simulink library "maddogLibrary"  (R2012b)
settings: Solver=ode45  StartTime=0.0  StopTime=10.0  RelTol=1e-3
libraries: xbsIndex_r4 x208, maddogLibrary x2
settings Model: Creator=tmadden  LastModifiedBy=tmadden

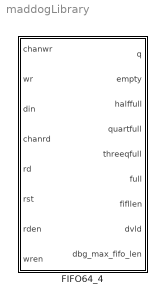
== system maddogLibrary ==
  FIFO64_4 : Subsystem  mask{fifo_len_p2=9}
      mask prompts: fifo_len_p2 "Fifo Len, (enter 8 for 256)"

== system maddogLibrary/FIFO64_4 ==
  chanwr : Inport
  wr : Inport  Port=2
  din : Inport  Port=3
  chanrd : Inport  Port=4
  rd : Inport  Port=5
  rst : Inport  Port=6
  rden : Inport  Port=7
  wren : Inport  Port=8
  FIFO32_1 : maddogLibrary/FIFO64_4/FIFO32_2
  FIFO32_2 : Subsystem
  Subsystem1 : Subsystem
  Subsystem2 : Subsystem
  q : Outport
  empty : Outport  Port=2
  halffull : Outport  Port=3
  quartfull : Outport  Port=4
  threeqfull : Outport  Port=5
  full : Outport  Port=6
  fifllen : Outport  Port=7
  dvld : Outport  Port=8
  dbg_max_fifo_len : Outport  Port=9
  wires:
  wr/1 -> FIFO32_1/2, FIFO32_2/2(wr)
  rst/1 -> FIFO32_1/6, FIFO32_2/6(rst)
  chanrd/1 -> Subsystem2/2(chanrd), Subsystem1/4(In4), FIFO32_1/4, FIFO32_2/4(chanrd)
  din/1 -> FIFO32_1/3, FIFO32_2/3(din)
  chanwr/1 -> Subsystem2/1(chanwr), FIFO32_1/1, FIFO32_2/1(chanwr)
  rd/1 -> FIFO32_1/5, FIFO32_2/5(rd)
  FIFO32_2/1(q) -> Subsystem1/1(In1)
  FIFO32_2/2(empty) -> Subsystem1/2(In2)
  FIFO32_2/3(halffull) -> Subsystem1/3(In3)
  FIFO32_2/4(quartfull) -> Subsystem1/5(In5)
  FIFO32_2/5(threeqfull) -> Subsystem1/6(In6)
  FIFO32_2/6(full) -> Subsystem1/7(In7)
  FIFO32_2/7(fifllen) -> Subsystem1/8(In8)
  FIFO32_2/8(dvld) -> Subsystem1/9(In9)
  FIFO32_1/1 -> Subsystem1/10(In10)
  FIFO32_1/2 -> Subsystem1/11(In11)
  FIFO32_1/3 -> Subsystem1/12(In12)
  FIFO32_1/4 -> Subsystem1/13(In13)
  FIFO32_1/5 -> Subsystem1/14(In14)
  FIFO32_1/6 -> Subsystem1/15(In15)
  FIFO32_1/8 -> Subsystem1/17(In17)
  Subsystem1/1(Out1) -> q/1
  Subsystem1/2(Out2) -> empty/1
  Subsystem1/3(Out3) -> halffull/1
  Subsystem1/4(Out4) -> quartfull/1
  Subsystem1/5(Out5) -> threeqfull/1
  Subsystem1/6(Out6) -> full/1
  Subsystem1/7(Out7) -> fifllen/1
  Subsystem1/8(Out8) -> dvld/1
  rden/1 -> Subsystem2/3(rden)
  wren/1 -> Subsystem2/4(wren)
  Subsystem2/2(rdl) -> FIFO32_2/7(rden)
  Subsystem2/3(wrh) -> FIFO32_1/8
  Subsystem2/1(wrl) -> FIFO32_2/8(wren)
  Subsystem2/4(rdh) -> FIFO32_1/7
  FIFO32_1/7 -> Subsystem1/16(In16)
  FIFO32_1/9 -> dbg_max_fifo_len/1

== system maddogLibrary/FIFO64_4/FIFO32_2 ==
  chanwr : Inport
  wr : Inport  Port=2
  din : Inport  Port=3
  chanrd : Inport  Port=4
  rd : Inport  Port=5
  rst : Inport  Port=6
  rden : Inport  Port=7
  wren : Inport  Port=8
  FIFO16Cir_1 : Subsystem
  FIFO16Cir_2 : maddogLibrary/FIFO64_4/FIFO32_2/FIFO16Cir_1
  Subsystem : Subsystem
  Subsystem1 : Subsystem
  q : Outport
  empty : Outport  Port=2
  halffull : Outport  Port=3
  quartfull : Outport  Port=4
  threeqfull : Outport  Port=5
  full : Outport  Port=6
  fifllen : Outport  Port=7
  dvld : Outport  Port=8
  dbg_max_fifo_len : Outport  Port=9
  wires:
  wr/1 -> FIFO16Cir_2/2, FIFO16Cir_1/2(wr)
  rst/1 -> FIFO16Cir_2/6, FIFO16Cir_1/6(rst)
  chanrd/1 -> Subsystem/2(chanrd), Subsystem1/4(In4), FIFO16Cir_2/4, FIFO16Cir_1/4(chanrd)
  din/1 -> FIFO16Cir_2/3, FIFO16Cir_1/3(din)
  chanwr/1 -> Subsystem/1(chanwr), FIFO16Cir_2/1, FIFO16Cir_1/1(chanwr)
  rd/1 -> FIFO16Cir_2/5, FIFO16Cir_1/5(rd)
  Subsystem/2(rdl) -> FIFO16Cir_1/7(rden)
  Subsystem/1(wrl) -> FIFO16Cir_1/8(wren)
  Subsystem/4(rdh) -> FIFO16Cir_2/7
  Subsystem/3(wrh) -> FIFO16Cir_2/8
  FIFO16Cir_1/1(q) -> Subsystem1/1(In1)
  FIFO16Cir_1/2(empty) -> Subsystem1/2(In2)
  FIFO16Cir_1/3(halffull) -> Subsystem1/3(In3)
  FIFO16Cir_1/4(quartfill) -> Subsystem1/5(In5)
  FIFO16Cir_1/5(threequartfull) -> Subsystem1/6(In6)
  FIFO16Cir_1/6(full) -> Subsystem1/7(In7)
  FIFO16Cir_1/7(fifolen) -> Subsystem1/8(In8)
  FIFO16Cir_1/8(dvld_out) -> Subsystem1/9(In9)
  FIFO16Cir_2/1 -> Subsystem1/10(In10)
  FIFO16Cir_2/2 -> Subsystem1/11(In11)
  FIFO16Cir_2/3 -> Subsystem1/12(In12)
  FIFO16Cir_2/4 -> Subsystem1/13(In13)
  FIFO16Cir_2/5 -> Subsystem1/14(In14)
  FIFO16Cir_2/6 -> Subsystem1/15(In15)
  FIFO16Cir_2/7 -> Subsystem1/16(In16)
  FIFO16Cir_2/8 -> Subsystem1/17(In17)
  Subsystem1/1(Out1) -> q/1
  Subsystem1/2(Out2) -> empty/1
  Subsystem1/3(Out3) -> halffull/1
  Subsystem1/4(Out4) -> quartfull/1
  Subsystem1/5(Out5) -> threeqfull/1
  Subsystem1/6(Out6) -> full/1
  Subsystem1/7(Out7) -> fifllen/1
  Subsystem1/8(Out8) -> dvld/1
  rden/1 -> Subsystem/3(rden)
  wren/1 -> Subsystem/4(wren)
  FIFO16Cir_2/9 -> dbg_max_fifo_len/1

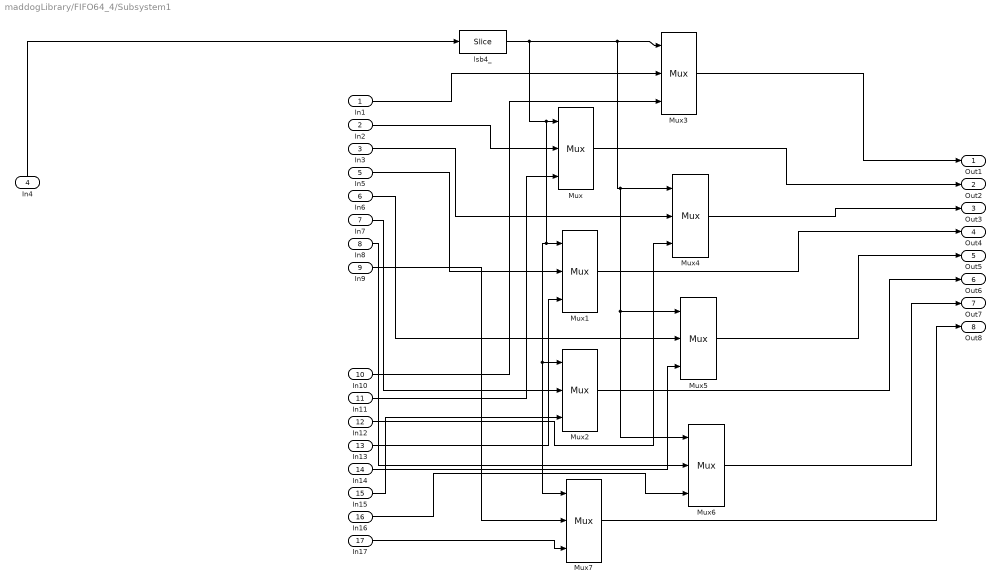
== system maddogLibrary/FIFO64_4/Subsystem1 ==
  In1 : Inport
  In2 : Inport  Port=2
  In3 : Inport  Port=3
  In4 : Inport  Port=4
  In5 : Inport  Port=5
  In6 : Inport  Port=6
  In7 : Inport  Port=7
  In8 : Inport  Port=8
  In9 : Inport  Port=9
  In10 : Inport  Port=10
  In11 : Inport  Port=11
  In12 : Inport  Port=12
  In13 : Inport  Port=13
  In14 : Inport  Port=14
  In15 : Inport  Port=15
  In16 : Inport  Port=16
  In17 : Inport  Port=17
  Mux{,1..7} (8 alike) : xbsIndex_r4/Mux  inputs=2  en=off  latency=0  precision=Full  arith_type=Unsigned  n_bits=16  bin_pt=14  quantization=Truncate  overflow=Wrap  dbl_ovrd=off  block_type=mux
  lsb4_ : xbsIndex_r4/Slice  nbits=1  boolean_output=on  mode=Lower Bit Location + Width  bit1=0  base1=MSB of Input  bit0=5  base0=LSB of Input  dbl_ovrd=off  block_type=slice
  Out1 : Outport
  Out2 : Outport  Port=2
  Out3 : Outport  Port=3
  Out4 : Outport  Port=4
  Out5 : Outport  Port=5
  Out6 : Outport  Port=6
  Out7 : Outport  Port=7
  Out8 : Outport  Port=8
  wires:
  In9/1 -> Mux7/2
  Mux3/1 -> Out1/1
  In11/1 -> Mux/3
  Mux7/1 -> Out8/1
  Mux1/1 -> Out4/1
  Mux5/1 -> Out5/1
  In17/1 -> Mux7/3
  Mux6/1 -> Out7/1
  In8/1 -> Mux6/2
  In10/1 -> Mux3/3
  In3/1 -> Mux4/2
  In13/1 -> Mux1/3
  In14/1 -> Mux5/3
  Mux4/1 -> Out3/1
  lsb4_/1 -> Mux7/1, Mux2/1, Mux1/1, Mux/1, Mux6/1, Mux5/1, Mux4/1, Mux3/1
  In4/1 -> lsb4_/1
  In12/1 -> Mux4/3
  In16/1 -> Mux6/3
  Mux2/1 -> Out6/1
  In15/1 -> Mux2/3
  In1/1 -> Mux3/2
  In6/1 -> Mux5/2
  In5/1 -> Mux1/2
  Mux/1 -> Out2/1
  In7/1 -> Mux2/2
  In2/1 -> Mux/2

== system maddogLibrary/FIFO64_4/Subsystem2 ==
  chanwr : Inport
  chanrd : Inport  Port=2
  rden : Inport  Port=3
  wren : Inport  Port=4
  Inverter : xbsIndex_r4/Inverter  en=off  latency=0  dbl_ovrd=off  block_type=inv
  Inverter1 : xbsIndex_r4/Inverter  en=off  latency=0  dbl_ovrd=off  block_type=inv
  Logical{1..4} (4 alike) : xbsIndex_r4/Logical  logical_function=AND  inputs=2  en=off  latency=0  precision=Full  arith_type=Unsigned  n_bits=16  bin_pt=0  align_bp=on  dbl_ovrd=off  block_type=logical
  lsb4_ : xbsIndex_r4/Slice  nbits=1  boolean_output=on  mode=Lower Bit Location + Width  bit1=0  base1=MSB of Input  bit0=5  base0=LSB of Input  dbl_ovrd=off  block_type=slice
  lsb4_1 : xbsIndex_r4/Slice  nbits=1  boolean_output=on  mode=Lower Bit Location + Width  bit1=0  base1=MSB of Input  bit0=5  base0=LSB of Input  dbl_ovrd=off  block_type=slice
  wrl : Outport
  rdl : Outport  Port=2
  wrh : Outport  Port=3
  rdh : Outport  Port=4
  wires:
  lsb4_/1 -> Logical2/1, Inverter/1
  lsb4_1/1 -> Logical1/1, Inverter1/1
  Inverter/1 -> Logical3/1
  Inverter1/1 -> Logical4/1
  chanrd/1 -> lsb4_1/1
  chanwr/1 -> lsb4_/1
  Logical1/1 -> rdh/1
  Logical2/1 -> wrh/1
  Logical3/1 -> wrl/1
  Logical4/1 -> rdl/1
  rden/1 -> Logical4/2, Logical1/2
  wren/1 -> Logical3/2, Logical2/2

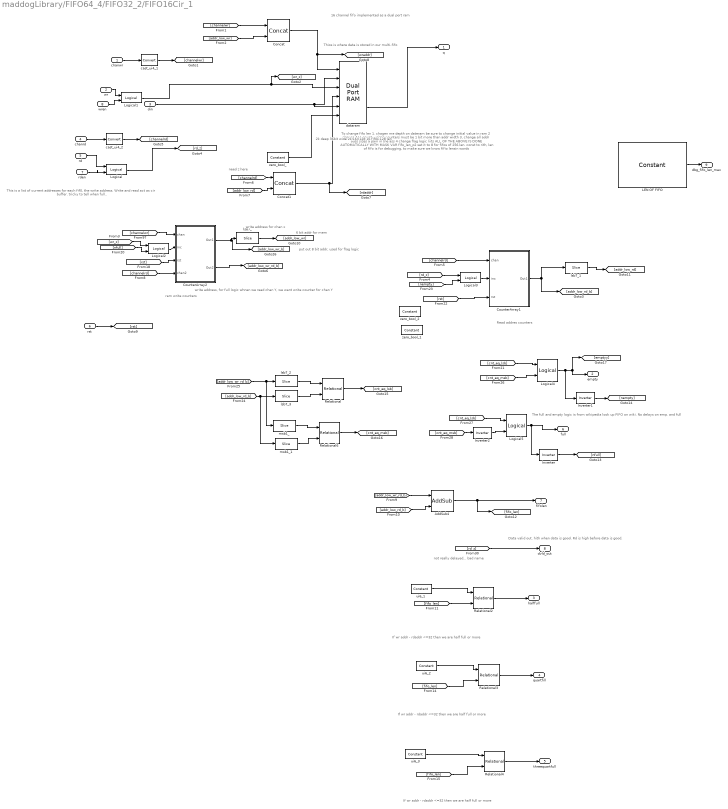
== system maddogLibrary/FIFO64_4/FIFO32_2/FIFO16Cir_1 ==
  note: The full and empty logic is from wikipedia
      | look up FIFO on wiki.
      | No delays on emp. and full
  note: not really delayed... bad name
  note: Data valid out.
      | hith when data is good.
      | Rd is high before data is good.
  note: 6 bit addr for mem
  note: put out 8 bit addr, used for flag logic
  note: To change fifo len
      | 1. chagen me depth on dateram
      | be sure to change initial value in ram
      | 2 change ALL counter sizes
      | counters must be 1 bit more than addr width
      | 3, change all addr buss sizes
      | a pain in the ass
      | 4 change flag logic liits
      |
      |
      | ALL OF THE ABOVE IS DONE
      | AUTOMATICALLY
      | WITH MASK VAR
      | fifo_len_p2
      | set it to 8 for fifos of 256 len.
      | const to rith, len of fifo
      | is for debugging, to make sure we know fifio lensin words
  note: 2k deep
      | 36bit wide
      | 2k/16=128
      | 16 fif0s,128 len
  note: If wr addr - rdaddr <=32 then we are half full or more
  note: ram write counters
  note: write address, for full logic
      | whnen we read chan Y,
      | we want write counter for chan Y
  note: write address for chan x
  note: need z here
  note: This is a list of current addresses for each fif0, the write address.
      | Write and read act as cir buffer. tricky to tell when full..
  note: Thios is where data is stored in our multi-fifo
  note: 16 channel fifo implemented as a dual port ram
  note: Read addres counters
  note: If wr addr - rdaddr <=32 then we are half full or more
  note: If wr addr - rdaddr <=32 then we are half full or more
  chanwr : Inport
  wr : Inport  Port=2
  din : Inport  Port=3
  chanrd : Inport  Port=4
  rd : Inport  Port=5
  rst : Inport  Port=6
  rden : Inport  Port=7
  wren : Inport  Port=8
  AddSub4 : xbsIndex_r4/AddSub  mode=Subtraction  use_carryin=off  use_carryout=off  en=off  latency=0  precision=User Defined  arith_type=Unsigned  n_bits=8  bin_pt=0  quantization=Truncate  overflow=Wrap  dbl_ovrd=off  use_behavioral_HDL=off  hw_selection=Fabric  pipelined=off  block_type=addsub
  Concat : xbsIndex_r4/Concat  num_inputs=2  dbl_ovrd=off  block_type=concat
  Concat1 : xbsIndex_r4/Concat  num_inputs=2  dbl_ovrd=off  block_type=concat
  CounterArray1 : Subsystem
  CounterArray2 : Subsystem
  Inverter : xbsIndex_r4/Inverter  en=off  latency=0  dbl_ovrd=off  block_type=inv
  Inverter1 : xbsIndex_r4/Inverter  en=off  latency=0  dbl_ovrd=off  block_type=inv
  Inverter2 : xbsIndex_r4/Inverter  en=off  latency=0  dbl_ovrd=off  block_type=inv
  LEN OF FIFO : xbsIndex_r4/Constant  const=2^fifo_len_p2  gui_display_data_type=Fixed-point  arith_type=Unsigned  n_bits=fifo_len_p2+1  bin_pt=0  preci_type=Single  exp_width=8  frac_width=24  explicit_period=on  period=1  equ=P=C  opselect=C  inp2=PCIN>>17  opr=+  inp1=P  carry=CIN  dbl_ovrd=off  block_type=constant
  Logical{,1..5} (6 alike) : xbsIndex_r4/Logical  logical_function=AND  inputs=2  en=off  latency=0  precision=Full  arith_type=Unsigned  n_bits=16  bin_pt=0  align_bp=on  dbl_ovrd=off  block_type=logical
  Relational : xbsIndex_r4/Relational  mode=a=b  en=off  latency=0  dbl_ovrd=off  block_type=relational
  Relational2 : xbsIndex_r4/Relational  mode=a<=b  en=off  latency=1  dbl_ovrd=off  block_type=relational
  Relational3 : xbsIndex_r4/Relational  mode=a<=b  en=off  latency=1  dbl_ovrd=off  block_type=relational
  Relational4 : xbsIndex_r4/Relational  mode=a<=b  en=off  latency=1  dbl_ovrd=off  block_type=relational
  Relational6 : xbsIndex_r4/Relational  mode=a=b  en=off  latency=0  dbl_ovrd=off  block_type=relational
  cast_ui4_1 : xbsIndex_r4/Convert  gui_display_data_type=Fixed-point  arith_type=Unsigned  n_bits=4  bin_pt=0  float_type=Single  exp_bits=8  fraction_bits=24  quantization=Truncate  overflow=Wrap  en=off  latency=0  dbl_ovrd=off  pipeline=off  block_type=convert
  cast_ui4_2 : xbsIndex_r4/Convert  gui_display_data_type=Fixed-point  arith_type=Unsigned  n_bits=4  bin_pt=0  float_type=Single  exp_bits=8  fraction_bits=24  quantization=Truncate  overflow=Wrap  en=off  latency=0  dbl_ovrd=off  pipeline=off  block_type=convert
  dataram : xbsIndex_r4/Dual Port RAM  depth=16 * (2^(fifo_len_p2))  initVector="zeros(1,16* 2^(fifo_len_p2)  )"  distributed_mem=Block RAM  init_a=0  init_b=0  rst_a=off  rst_b=off  en_a=off  en_b=off  latency=1  write_mode_A=Read Before Write  write_mode_B=Read After Write  dbl_ovrd=off  optimize=Area  block_type=dpram
  lsb7_{,1..3} (4 alike) : xbsIndex_r4/Slice  nbits=fifo_len_p2  boolean_output=off  mode=Lower Bit Location + Width  bit1=0  base1=MSB of Input  bit0=0  base0=LSB of Input  dbl_ovrd=off  block_type=slice
  msb1_ : xbsIndex_r4/Slice  nbits=1  boolean_output=off  mode=Upper Bit Location + Width  bit1=0  base1=MSB of Input  bit0=0  base0=LSB of Input  dbl_ovrd=off  block_type=slice
  msb1_1 : xbsIndex_r4/Slice  nbits=1  boolean_output=off  mode=Upper Bit Location + Width  bit1=0  base1=MSB of Input  bit0=0  base0=LSB of Input  dbl_ovrd=off  block_type=slice
  ui6_1 : xbsIndex_r4/Constant  const=(2^fifo_len_p2) / 2  gui_display_data_type=Fixed-point  arith_type=Unsigned  n_bits=fifo_len_p2  bin_pt=0  preci_type=Single  exp_width=8  frac_width=24  explicit_period=on  period=1  equ=P=C  opselect=C  inp2=PCIN>>17  opr=+  inp1=P  carry=CIN  dbl_ovrd=off  block_type=constant
  ui6_2 : xbsIndex_r4/Constant  const=(2^fifo_len_p2) / 4  gui_display_data_type=Fixed-point  arith_type=Unsigned  n_bits=fifo_len_p2  bin_pt=0  preci_type=Single  exp_width=8  frac_width=24  explicit_period=on  period=1  equ=P=C  opselect=C  inp2=PCIN>>17  opr=+  inp1=P  carry=CIN  dbl_ovrd=off  block_type=constant
  ui6_3 : xbsIndex_r4/Constant  const=(3*(2^fifo_len_p2)) / 4  gui_display_data_type=Fixed-point  arith_type=Unsigned  n_bits=fifo_len_p2  bin_pt=0  preci_type=Single  exp_width=8  frac_width=24  explicit_period=on  period=1  equ=P=C  opselect=C  inp2=PCIN>>17  opr=+  inp1=P  carry=CIN  dbl_ovrd=off  block_type=constant
  zero_bool_ : xbsIndex_r4/Constant  const=0  gui_display_data_type=Boolean  arith_type=Boolean  n_bits=36  bin_pt=0  preci_type=Single  exp_width=8  frac_width=24  explicit_period=on  period=1  equ=P=C  opselect=C  inp2=PCIN>>17  opr=+  inp1=P  carry=CIN  dbl_ovrd=off  block_type=constant
  zero_bool_1 : xbsIndex_r4/Constant  const=0  gui_display_data_type=Boolean  arith_type=Boolean  n_bits=36  bin_pt=0  preci_type=Single  exp_width=8  frac_width=24  explicit_period=on  period=1  equ=P=C  opselect=C  inp2=PCIN>>17  opr=+  inp1=P  carry=CIN  dbl_ovrd=off  block_type=constant
  zero_bool_2 : xbsIndex_r4/Constant  const=0  gui_display_data_type=Boolean  arith_type=Boolean  n_bits=36  bin_pt=0  preci_type=Single  exp_width=8  frac_width=24  explicit_period=on  period=1  equ=P=C  opselect=C  inp2=PCIN>>17  opr=+  inp1=P  carry=CIN  dbl_ovrd=off  block_type=constant
  q : Outport
  empty : Outport  Port=2
  halffull : Outport  Port=3
  quartfill : Outport  Port=4
  threequartfull : Outport  Port=5
  full : Outport  Port=6
  fifolen : Outport  Port=7
  dvld_out : Outport  Port=8
  dbg_fifo_len_max : Outport  Port=9
  wires:
  chanwr/1 -> cast_ui4_1/1
  cast_ui4_1/1 -> [channelwr]
  [channelwr] -> Concat/1
  [addr_low_wr] -> Concat/2
  Concat/1 -> [wraddr], dataram/1
  Logical1/1 -> [wr_z], dataram/3
  din/1 -> dataram/5, dataram/2
  Logical/1 -> [rd_z]
  cast_ui4_2/1 -> [channelrd]
  chanrd/1 -> cast_ui4_2/1
  [channelrd] -> Concat1/1
  [addr_low_rd] -> Concat1/2
  Concat1/1 -> [rdaddr], dataram/4
  zero_bool_/1 -> dataram/6
  dataram/2 -> q/1
  [channelwr] -> CounterArray2/1(chan)
  CounterArray2/1(Out1) -> lsb7_/1, [addr_low_wr_b]
  [channelrd] -> CounterArray1/1(chan)
  CounterArray1/1(Out1) -> [addr_low_rd_b], lsb7_1/1
  [channelrd] -> CounterArray2/4(chan2)
  ui6_1/1 -> Relational2/1
  Relational2/1 -> halffull/1
  rst/1 -> [rst]
  [rst] -> CounterArray2/3(rst)
  [rst] -> CounterArray1/3(rst)
  rd/1 -> Logical/1
  rden/1 -> Logical/2
  wr/1 -> Logical1/1
  wren/1 -> Logical1/2
  ui6_2/1 -> Relational3/1
  Relational3/1 -> quartfill/1
  ui6_3/1 -> Relational4/1
  Relational4/1 -> threequartfull/1
  CounterArray2/2(Out2) -> [addr_low_wr_rd_b]
  lsb7_/1 -> [addr_low_wr]
  lsb7_1/1 -> [addr_low_rd]
  [addr_low_wr_rd_b] -> AddSub4/1
  AddSub4/1 -> fifolen/1, [fifo_len]
  [addr_low_rd_b] -> AddSub4/2
  [fifo_len] -> Relational2/2
  [fifo_len] -> Relational3/2
  [fifo_len] -> Relational4/2
  Logical2/1 -> CounterArray2/2(inc)
  [wr_z] -> Logical2/1
  Inverter/1 -> [nfull]
  [nfull] -> Logical2/2
  Logical3/1 -> CounterArray1/2(inc)
  [rd_z] -> Logical3/1
  Inverter1/1 -> [nempty]
  [nempty] -> Logical3/2
  [addr_low_wr_rd_b] -> msb1_/1, lsb7_2/1
  [addr_low_rd_b] -> msb1_1/1, lsb7_3/1
  lsb7_2/1 -> Relational/1
  lsb7_3/1 -> Relational/2
  msb1_/1 -> Relational6/1
  msb1_1/1 -> Relational6/2
  Relational/1 -> [cnt_eq_lsb]
  Relational6/1 -> [cnt_eq_msb]
  [cnt_eq_lsb] -> Logical4/1
  [cnt_eq_msb] -> Logical4/2
  Logical4/1 -> Inverter1/1, empty/1, [emptyy]
  [cnt_eq_lsb] -> Logical5/1
  [cnt_eq_msb] -> Inverter2/1
  Logical5/1 -> Inverter/1, full/1
  Inverter2/1 -> Logical5/2
  [rd_z] -> dvld_out/1
  LEN OF FIFO/1 -> dbg_fifo_len_max/1

== system maddogLibrary/FIFO64_4/FIFO32_2/Subsystem ==
  chanwr : Inport
  chanrd : Inport  Port=2
  rden : Inport  Port=3
  wren : Inport  Port=4
  Inverter : xbsIndex_r4/Inverter  en=off  latency=0  dbl_ovrd=off  block_type=inv
  Inverter1 : xbsIndex_r4/Inverter  en=off  latency=0  dbl_ovrd=off  block_type=inv
  Logical{1..4} (4 alike) : xbsIndex_r4/Logical  logical_function=AND  inputs=2  en=off  latency=0  precision=Full  arith_type=Unsigned  n_bits=16  bin_pt=0  align_bp=on  dbl_ovrd=off  block_type=logical
  lsb4_ : xbsIndex_r4/Slice  nbits=1  boolean_output=on  mode=Lower Bit Location + Width  bit1=0  base1=MSB of Input  bit0=4  base0=LSB of Input  dbl_ovrd=off  block_type=slice
  lsb4_1 : xbsIndex_r4/Slice  nbits=1  boolean_output=on  mode=Lower Bit Location + Width  bit1=0  base1=MSB of Input  bit0=4  base0=LSB of Input  dbl_ovrd=off  block_type=slice
  wrl : Outport
  rdl : Outport  Port=2
  wrh : Outport  Port=3
  rdh : Outport  Port=4
  wires:
  lsb4_/1 -> Logical2/1, Inverter/1
  lsb4_1/1 -> Logical1/1, Inverter1/1
  Inverter/1 -> Logical3/1
  Inverter1/1 -> Logical4/1
  chanrd/1 -> lsb4_1/1
  chanwr/1 -> lsb4_/1
  Logical1/1 -> rdh/1
  Logical2/1 -> wrh/1
  Logical3/1 -> wrl/1
  Logical4/1 -> rdl/1
  rden/1 -> Logical4/2, Logical1/2
  wren/1 -> Logical3/2, Logical2/2

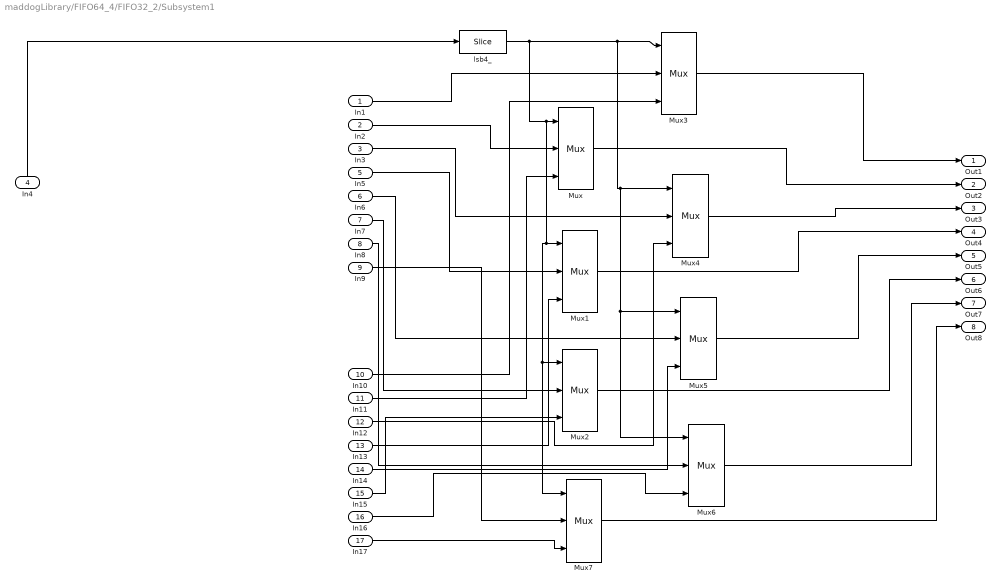
== system maddogLibrary/FIFO64_4/FIFO32_2/Subsystem1 ==
  In1 : Inport
  In2 : Inport  Port=2
  In3 : Inport  Port=3
  In4 : Inport  Port=4
  In5 : Inport  Port=5
  In6 : Inport  Port=6
  In7 : Inport  Port=7
  In8 : Inport  Port=8
  In9 : Inport  Port=9
  In10 : Inport  Port=10
  In11 : Inport  Port=11
  In12 : Inport  Port=12
  In13 : Inport  Port=13
  In14 : Inport  Port=14
  In15 : Inport  Port=15
  In16 : Inport  Port=16
  In17 : Inport  Port=17
  Mux{,1..7} (8 alike) : xbsIndex_r4/Mux  inputs=2  en=off  latency=0  precision=Full  arith_type=Unsigned  n_bits=16  bin_pt=14  quantization=Truncate  overflow=Wrap  dbl_ovrd=off  block_type=mux
  lsb4_ : xbsIndex_r4/Slice  nbits=1  boolean_output=on  mode=Lower Bit Location + Width  bit1=0  base1=MSB of Input  bit0=4  base0=LSB of Input  dbl_ovrd=off  block_type=slice
  Out1 : Outport
  Out2 : Outport  Port=2
  Out3 : Outport  Port=3
  Out4 : Outport  Port=4
  Out5 : Outport  Port=5
  Out6 : Outport  Port=6
  Out7 : Outport  Port=7
  Out8 : Outport  Port=8
  wires:
  In9/1 -> Mux7/2
  Mux3/1 -> Out1/1
  In11/1 -> Mux/3
  Mux7/1 -> Out8/1
  Mux1/1 -> Out4/1
  Mux5/1 -> Out5/1
  In17/1 -> Mux7/3
  Mux6/1 -> Out7/1
  In8/1 -> Mux6/2
  In10/1 -> Mux3/3
  In3/1 -> Mux4/2
  In13/1 -> Mux1/3
  In14/1 -> Mux5/3
  Mux4/1 -> Out3/1
  lsb4_/1 -> Mux7/1, Mux2/1, Mux1/1, Mux/1, Mux6/1, Mux5/1, Mux4/1, Mux3/1
  In4/1 -> lsb4_/1
  In12/1 -> Mux4/3
  In16/1 -> Mux6/3
  Mux2/1 -> Out6/1
  In15/1 -> Mux2/3
  In1/1 -> Mux3/2
  In6/1 -> Mux5/2
  In5/1 -> Mux1/2
  Mux/1 -> Out2/1
  In7/1 -> Mux2/2
  In2/1 -> Mux/2

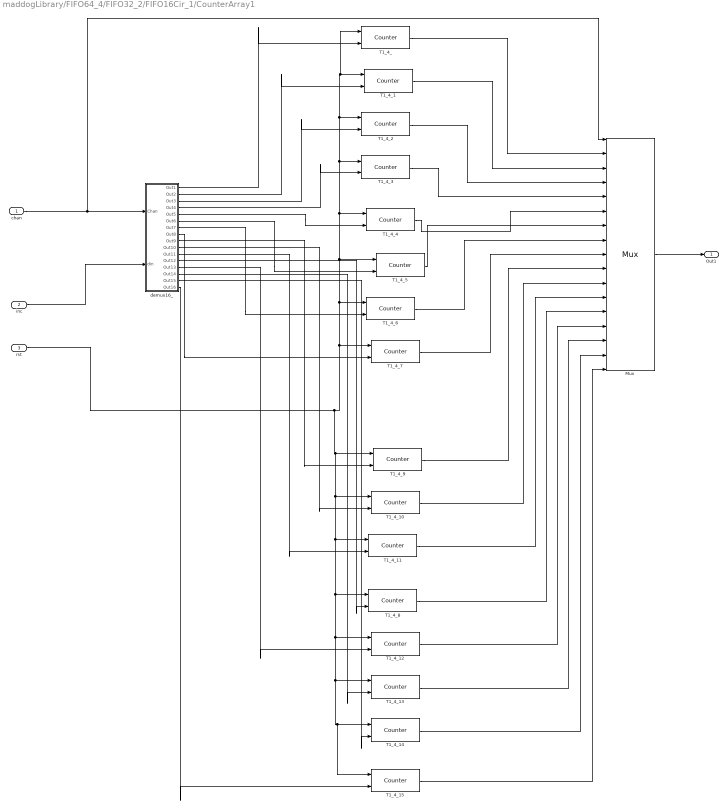
== system maddogLibrary/FIFO64_4/FIFO32_2/FIFO16Cir_1/CounterArray1 ==
  chan : Inport
  inc : Inport  Port=2
  rst : Inport  Port=3
  Mux : xbsIndex_r4/Mux  inputs=16  en=off  latency=0  precision=Full  arith_type=Unsigned  n_bits=16  bin_pt=14  quantization=Truncate  overflow=Wrap  dbl_ovrd=off  block_type=mux
  T1_4_{,1..15} (16 alike) : xbsIndex_r4/Counter  cnt_type=Free Running  cnt_to=Inf  operation=Up  start_count=0  cnt_by_val=1  arith_type=Unsigned  n_bits=1+fifo_len_p2  bin_pt=0  load_pin=off  rst=on  en=on  explicit_period=on  period=1  dbl_ovrd=off  use_behavioral_HDL=off  implementation=Fabric  block_type=counter
  demux16_ : Subsystem
  Out1 : Outport
  wires:
  chan/1 -> Mux/1, demux16_/1(Chan)
  inc/1 -> demux16_/2(din)
  rst/1 -> T1_4_9/1, T1_4_10/1, T1_4_11/1, T1_4_8/1, T1_4_12/1, T1_4_13/1, T1_4_14/1, T1_4_15/1, T1_4_7/1, T1_4_6/1, T1_4_5/1, T1_4_3/1, T1_4_2/1, T1_4_1/1, T1_4_/1, T1_4_4/1
  demux16_/1(Out1) -> T1_4_/2
  demux16_/2(Out2) -> T1_4_1/2
  demux16_/3(Out3) -> T1_4_2/2
  demux16_/4(Out4) -> T1_4_3/2
  demux16_/5(Out5) -> T1_4_4/2
  demux16_/6(Out6) -> T1_4_5/2
  demux16_/7(Out7) -> T1_4_6/2
  demux16_/8(Out8) -> T1_4_7/2
  demux16_/9(Out9) -> T1_4_9/2
  demux16_/10(Out10) -> T1_4_10/2
  demux16_/11(Out11) -> T1_4_11/2
  demux16_/12(Out12) -> T1_4_8/2
  demux16_/13(Out13) -> T1_4_12/2
  demux16_/14(Out14) -> T1_4_13/2
  demux16_/15(Out15) -> T1_4_14/2
  demux16_/16(Out16) -> T1_4_15/2
  T1_4_/1 -> Mux/2
  T1_4_1/1 -> Mux/3
  T1_4_2/1 -> Mux/4
  T1_4_3/1 -> Mux/5
  T1_4_4/1 -> Mux/6
  T1_4_5/1 -> Mux/7
  T1_4_6/1 -> Mux/8
  T1_4_7/1 -> Mux/9
  T1_4_9/1 -> Mux/10
  T1_4_10/1 -> Mux/11
  T1_4_11/1 -> Mux/12
  T1_4_8/1 -> Mux/13
  T1_4_12/1 -> Mux/14
  T1_4_13/1 -> Mux/15
  T1_4_14/1 -> Mux/16
  T1_4_15/1 -> Mux/17
  Mux/1 -> Out1/1

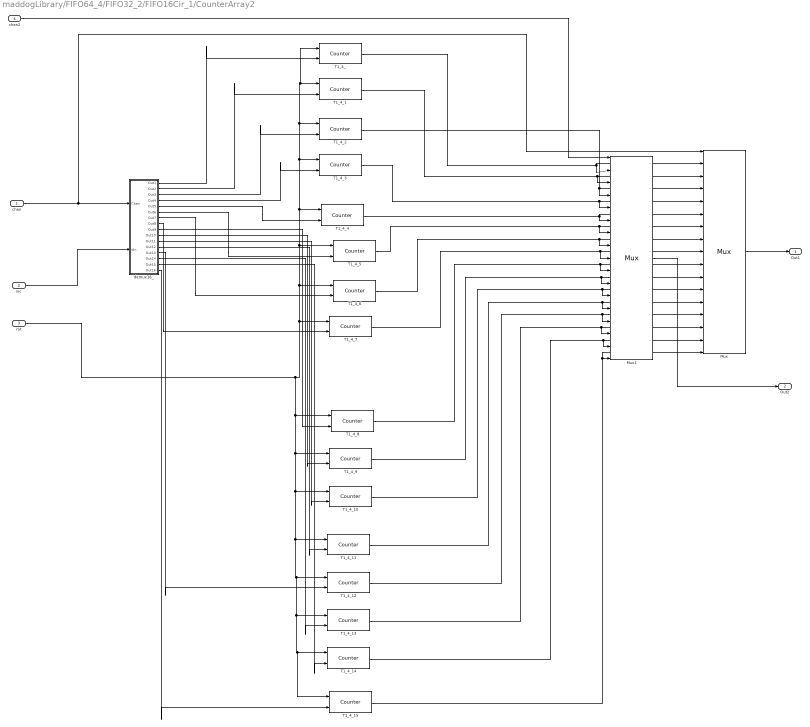
== system maddogLibrary/FIFO64_4/FIFO32_2/FIFO16Cir_1/CounterArray2 ==
  chan : Inport
  inc : Inport  Port=2
  rst : Inport  Port=3
  chan2 : Inport  Port=4
  Mux : xbsIndex_r4/Mux  inputs=16  en=off  latency=0  precision=Full  arith_type=Unsigned  n_bits=16  bin_pt=14  quantization=Truncate  overflow=Wrap  dbl_ovrd=off  block_type=mux
  Mux1 : xbsIndex_r4/Mux  inputs=16  en=off  latency=0  precision=Full  arith_type=Unsigned  n_bits=16  bin_pt=14  quantization=Truncate  overflow=Wrap  dbl_ovrd=off  block_type=mux
  T1_4_{,1..15} (16 alike) : xbsIndex_r4/Counter  cnt_type=Free Running  cnt_to=Inf  operation=Up  start_count=0  cnt_by_val=1  arith_type=Unsigned  n_bits=fifo_len_p2+1  bin_pt=0  load_pin=off  rst=on  en=on  explicit_period=on  period=1  dbl_ovrd=off  use_behavioral_HDL=off  implementation=Fabric  block_type=counter
  demux16_ : Subsystem
  Out1 : Outport
  Out2 : Outport  Port=2
  wires:
  chan/1 -> Mux/1, demux16_/1(Chan)
  inc/1 -> demux16_/2(din)
  rst/1 -> T1_4_8/1, T1_4_9/1, T1_4_10/1, T1_4_11/1, T1_4_12/1, T1_4_13/1, T1_4_14/1, T1_4_15/1, T1_4_7/1, T1_4_6/1, T1_4_5/1, T1_4_4/1, T1_4_3/1, T1_4_2/1, T1_4_1/1, T1_4_/1
  demux16_/1(Out1) -> T1_4_/2
  demux16_/2(Out2) -> T1_4_1/2
  demux16_/3(Out3) -> T1_4_2/2
  demux16_/4(Out4) -> T1_4_3/2
  demux16_/5(Out5) -> T1_4_4/2
  demux16_/6(Out6) -> T1_4_5/2
  demux16_/7(Out7) -> T1_4_6/2
  demux16_/8(Out8) -> T1_4_7/2
  demux16_/9(Out9) -> T1_4_8/2
  demux16_/10(Out10) -> T1_4_9/2
  demux16_/11(Out11) -> T1_4_10/2
  demux16_/12(Out12) -> T1_4_11/2
  demux16_/13(Out13) -> T1_4_12/2
  demux16_/14(Out14) -> T1_4_13/2
  demux16_/15(Out15) -> T1_4_14/2
  demux16_/16(Out16) -> T1_4_15/2
  T1_4_/1 -> Mux1/2, Mux/2
  T1_4_1/1 -> Mux1/3, Mux/3
  T1_4_2/1 -> Mux1/4, Mux/4
  T1_4_3/1 -> Mux1/5, Mux/5
  T1_4_4/1 -> Mux/6, Mux1/6
  T1_4_5/1 -> Mux1/7, Mux/7
  T1_4_6/1 -> Mux1/8, Mux/8
  T1_4_7/1 -> Mux1/9, Mux/9
  T1_4_8/1 -> Mux1/10, Mux/10
  T1_4_9/1 -> Mux1/11, Mux/11
  T1_4_10/1 -> Mux1/12, Mux/12
  T1_4_11/1 -> Mux1/13, Mux/13
  T1_4_12/1 -> Mux1/14, Mux/14
  T1_4_13/1 -> Mux1/15, Mux/15
  T1_4_14/1 -> Mux1/16, Mux/16
  T1_4_15/1 -> Mux/17, Mux1/17
  Mux/1 -> Out1/1
  chan2/1 -> Mux1/1
  Mux1/1 -> Out2/1

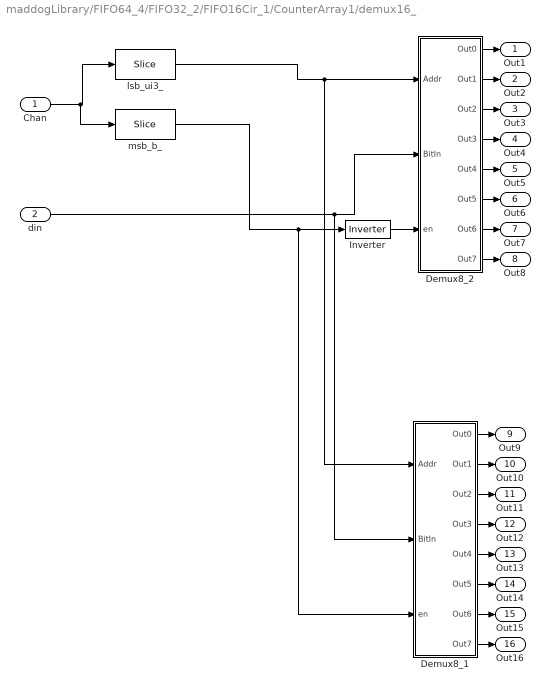
== system maddogLibrary/FIFO64_4/FIFO32_2/FIFO16Cir_1/CounterArray1/demux16_ ==
  Chan : Inport
  din : Inport  Port=2
  Demux8_1 : Subsystem
  Demux8_2 : Subsystem
  Inverter : xbsIndex_r4/Inverter  en=off  latency=0  dbl_ovrd=off  block_type=inv
  lsb_ui3_ : xbsIndex_r4/Slice  nbits=3  boolean_output=off  mode=Lower Bit Location + Width  bit1=0  base1=MSB of Input  bit0=0  base0=LSB of Input  dbl_ovrd=off  block_type=slice
  msb_b_ : xbsIndex_r4/Slice  nbits=1  boolean_output=on  mode=Upper Bit Location + Width  bit1=0  base1=MSB of Input  bit0=0  base0=LSB of Input  dbl_ovrd=off  block_type=slice
  Out1 : Outport
  Out2 : Outport  Port=2
  Out3 : Outport  Port=3
  Out4 : Outport  Port=4
  Out5 : Outport  Port=5
  Out6 : Outport  Port=6
  Out7 : Outport  Port=7
  Out8 : Outport  Port=8
  Out9 : Outport  Port=9
  Out10 : Outport  Port=10
  Out11 : Outport  Port=11
  Out12 : Outport  Port=12
  Out13 : Outport  Port=13
  Out14 : Outport  Port=14
  Out15 : Outport  Port=15
  Out16 : Outport  Port=16
  wires:
  Demux8_1/1(Out0) -> Out9/1
  Demux8_1/6(Out5) -> Out14/1
  Demux8_2/5(Out4) -> Out5/1
  Demux8_2/7(Out6) -> Out7/1
  Demux8_1/2(Out1) -> Out10/1
  Demux8_1/3(Out2) -> Out11/1
  Demux8_2/4(Out3) -> Out4/1
  Demux8_1/7(Out6) -> Out15/1
  Demux8_1/4(Out3) -> Out12/1
  Demux8_2/8(Out7) -> Out8/1
  Demux8_2/1(Out0) -> Out1/1
  Demux8_1/5(Out4) -> Out13/1
  Demux8_2/6(Out5) -> Out6/1
  Demux8_2/2(Out1) -> Out2/1
  Demux8_2/3(Out2) -> Out3/1
  Demux8_1/8(Out7) -> Out16/1
  Chan/1 -> msb_b_/1, lsb_ui3_/1
  lsb_ui3_/1 -> Demux8_1/1(Addr), Demux8_2/1(Addr)
  msb_b_/1 -> Demux8_1/3(en), Inverter/1
  din/1 -> Demux8_2/2(BitIn), Demux8_1/2(BitIn)
  Inverter/1 -> Demux8_2/3(en)

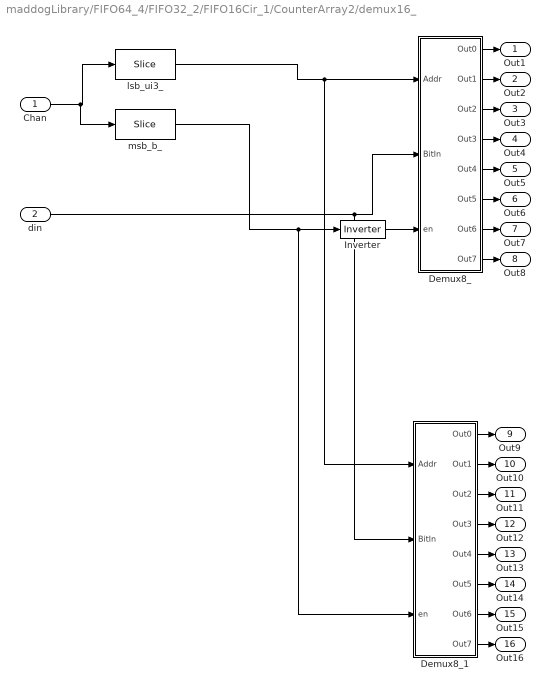
== system maddogLibrary/FIFO64_4/FIFO32_2/FIFO16Cir_1/CounterArray2/demux16_ ==
  Chan : Inport
  din : Inport  Port=2
  Demux8_ : Subsystem
  Demux8_1 : Subsystem
  Inverter : xbsIndex_r4/Inverter  en=off  latency=0  dbl_ovrd=off  block_type=inv
  lsb_ui3_ : xbsIndex_r4/Slice  nbits=3  boolean_output=off  mode=Lower Bit Location + Width  bit1=0  base1=MSB of Input  bit0=0  base0=LSB of Input  dbl_ovrd=off  block_type=slice
  msb_b_ : xbsIndex_r4/Slice  nbits=1  boolean_output=on  mode=Upper Bit Location + Width  bit1=0  base1=MSB of Input  bit0=0  base0=LSB of Input  dbl_ovrd=off  block_type=slice
  Out1 : Outport
  Out2 : Outport  Port=2
  Out3 : Outport  Port=3
  Out4 : Outport  Port=4
  Out5 : Outport  Port=5
  Out6 : Outport  Port=6
  Out7 : Outport  Port=7
  Out8 : Outport  Port=8
  Out9 : Outport  Port=9
  Out10 : Outport  Port=10
  Out11 : Outport  Port=11
  Out12 : Outport  Port=12
  Out13 : Outport  Port=13
  Out14 : Outport  Port=14
  Out15 : Outport  Port=15
  Out16 : Outport  Port=16
  wires:
  Demux8_1/1(Out0) -> Out9/1
  Demux8_1/6(Out5) -> Out14/1
  Demux8_/5(Out4) -> Out5/1
  Demux8_/7(Out6) -> Out7/1
  Demux8_1/2(Out1) -> Out10/1
  Demux8_1/3(Out2) -> Out11/1
  Demux8_/4(Out3) -> Out4/1
  Demux8_1/7(Out6) -> Out15/1
  Demux8_1/4(Out3) -> Out12/1
  Demux8_/8(Out7) -> Out8/1
  Demux8_/1(Out0) -> Out1/1
  Demux8_1/5(Out4) -> Out13/1
  Demux8_/6(Out5) -> Out6/1
  Demux8_/2(Out1) -> Out2/1
  Demux8_/3(Out2) -> Out3/1
  Demux8_1/8(Out7) -> Out16/1
  Chan/1 -> msb_b_/1, lsb_ui3_/1
  lsb_ui3_/1 -> Demux8_1/1(Addr), Demux8_/1(Addr)
  msb_b_/1 -> Demux8_1/3(en), Inverter/1
  din/1 -> Demux8_1/2(BitIn), Demux8_/2(BitIn)
  Inverter/1 -> Demux8_/3(en)

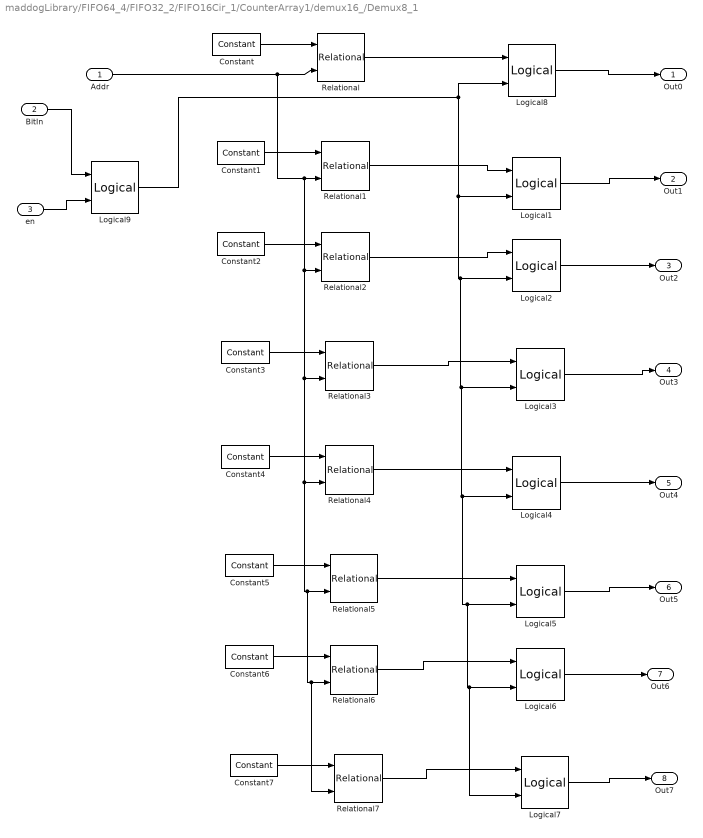
== system maddogLibrary/FIFO64_4/FIFO32_2/FIFO16Cir_1/CounterArray1/demux16_/Demux8_1 ==
  Addr : Inport
  BitIn : Inport  Port=2
  en : Inport  Port=3
  Constant : xbsIndex_r4/Constant  const=0  gui_display_data_type=Fixed-point  arith_type=Unsigned  n_bits=3  bin_pt=0  preci_type=Single  exp_width=8  frac_width=24  explicit_period=on  period=1  equ=P=C  opselect=C  inp2=PCIN>>17  opr=+  inp1=P  carry=CIN  dbl_ovrd=off  block_type=constant
  Constant1 : xbsIndex_r4/Constant  const=1  gui_display_data_type=Fixed-point  arith_type=Unsigned  n_bits=3  bin_pt=0  preci_type=Single  exp_width=8  frac_width=24  explicit_period=on  period=1  equ=P=C  opselect=C  inp2=PCIN>>17  opr=+  inp1=P  carry=CIN  dbl_ovrd=off  block_type=constant
  Constant2 : xbsIndex_r4/Constant  const=2  gui_display_data_type=Fixed-point  arith_type=Unsigned  n_bits=3  bin_pt=0  preci_type=Single  exp_width=8  frac_width=24  explicit_period=on  period=1  equ=P=C  opselect=C  inp2=PCIN>>17  opr=+  inp1=P  carry=CIN  dbl_ovrd=off  block_type=constant
  Constant3 : xbsIndex_r4/Constant  const=3  gui_display_data_type=Fixed-point  arith_type=Unsigned  n_bits=3  bin_pt=0  preci_type=Single  exp_width=8  frac_width=24  explicit_period=on  period=1  equ=P=C  opselect=C  inp2=PCIN>>17  opr=+  inp1=P  carry=CIN  dbl_ovrd=off  block_type=constant
  Constant4 : xbsIndex_r4/Constant  const=4  gui_display_data_type=Fixed-point  arith_type=Unsigned  n_bits=3  bin_pt=0  preci_type=Single  exp_width=8  frac_width=24  explicit_period=on  period=1  equ=P=C  opselect=C  inp2=PCIN>>17  opr=+  inp1=P  carry=CIN  dbl_ovrd=off  block_type=constant
  Constant5 : xbsIndex_r4/Constant  const=5  gui_display_data_type=Fixed-point  arith_type=Unsigned  n_bits=3  bin_pt=0  preci_type=Single  exp_width=8  frac_width=24  explicit_period=on  period=1  equ=P=C  opselect=C  inp2=PCIN>>17  opr=+  inp1=P  carry=CIN  dbl_ovrd=off  block_type=constant
  Constant6 : xbsIndex_r4/Constant  const=6  gui_display_data_type=Fixed-point  arith_type=Unsigned  n_bits=3  bin_pt=0  preci_type=Single  exp_width=8  frac_width=24  explicit_period=on  period=1  equ=P=C  opselect=C  inp2=PCIN>>17  opr=+  inp1=P  carry=CIN  dbl_ovrd=off  block_type=constant
  Constant7 : xbsIndex_r4/Constant  const=7  gui_display_data_type=Fixed-point  arith_type=Unsigned  n_bits=3  bin_pt=0  preci_type=Single  exp_width=8  frac_width=24  explicit_period=on  period=1  equ=P=C  opselect=C  inp2=PCIN>>17  opr=+  inp1=P  carry=CIN  dbl_ovrd=off  block_type=constant
  Logical{1..9} (9 alike) : xbsIndex_r4/Logical  logical_function=AND  inputs=2  en=off  latency=0  precision=Full  arith_type=Unsigned  n_bits=16  bin_pt=0  align_bp=on  dbl_ovrd=off  block_type=logical
  Relational{,1..7} (8 alike) : xbsIndex_r4/Relational  mode=a=b  en=off  latency=0  dbl_ovrd=off  block_type=relational
  Out0 : Outport
  Out1 : Outport  Port=2
  Out2 : Outport  Port=3
  Out3 : Outport  Port=4
  Out4 : Outport  Port=5
  Out5 : Outport  Port=6
  Out6 : Outport  Port=7
  Out7 : Outport  Port=8
  wires:
  Constant4/1 -> Relational4/1
  Constant5/1 -> Relational5/1
  Constant6/1 -> Relational6/1
  Constant1/1 -> Relational1/1
  Relational1/1 -> Logical1/1
  Relational2/1 -> Logical2/1
  Relational/1 -> Logical8/1
  Relational6/1 -> Logical6/1
  Relational3/1 -> Logical3/1
  Relational5/1 -> Logical5/1
  Relational4/1 -> Logical4/1
  Addr/1 -> Relational7/2, Relational6/2, Relational5/2, Relational4/2, Relational3/2, Relational2/2, Relational1/2, Relational/2
  Constant/1 -> Relational/1
  Constant2/1 -> Relational2/1
  Constant3/1 -> Relational3/1
  Constant7/1 -> Relational7/1
  Relational7/1 -> Logical7/1
  Logical9/1 -> Logical8/2, Logical1/2, Logical2/2, Logical3/2, Logical4/2, Logical5/2, Logical7/2, Logical6/2
  Logical8/1 -> Out0/1
  Logical1/1 -> Out1/1
  Logical2/1 -> Out2/1
  Logical3/1 -> Out3/1
  Logical4/1 -> Out4/1
  Logical5/1 -> Out5/1
  Logical6/1 -> Out6/1
  Logical7/1 -> Out7/1
  BitIn/1 -> Logical9/1
  en/1 -> Logical9/2

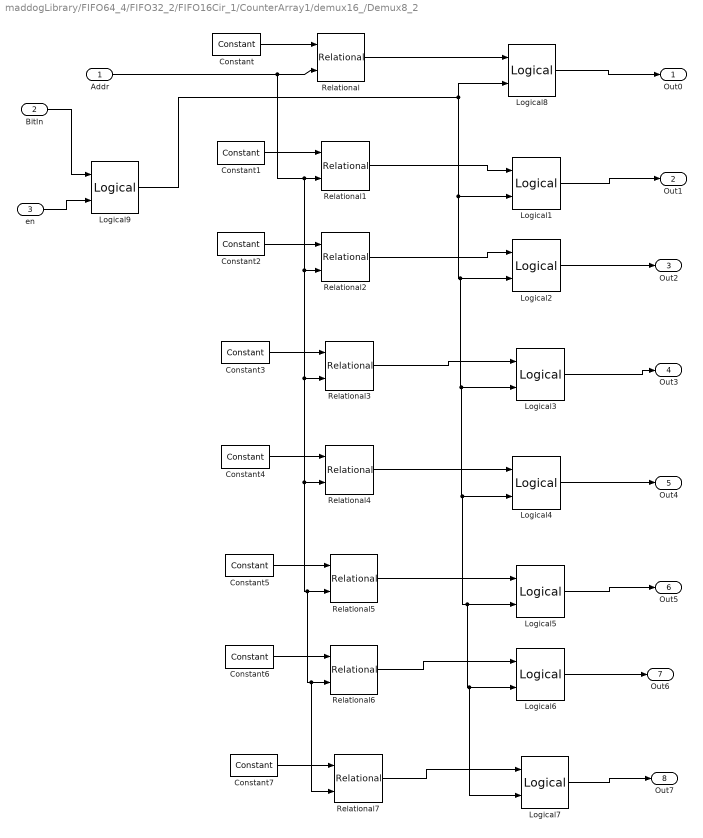
== system maddogLibrary/FIFO64_4/FIFO32_2/FIFO16Cir_1/CounterArray1/demux16_/Demux8_2 ==
  Addr : Inport
  BitIn : Inport  Port=2
  en : Inport  Port=3
  Constant : xbsIndex_r4/Constant  const=0  gui_display_data_type=Fixed-point  arith_type=Unsigned  n_bits=3  bin_pt=0  preci_type=Single  exp_width=8  frac_width=24  explicit_period=on  period=1  equ=P=C  opselect=C  inp2=PCIN>>17  opr=+  inp1=P  carry=CIN  dbl_ovrd=off  block_type=constant
  Constant1 : xbsIndex_r4/Constant  const=1  gui_display_data_type=Fixed-point  arith_type=Unsigned  n_bits=3  bin_pt=0  preci_type=Single  exp_width=8  frac_width=24  explicit_period=on  period=1  equ=P=C  opselect=C  inp2=PCIN>>17  opr=+  inp1=P  carry=CIN  dbl_ovrd=off  block_type=constant
  Constant2 : xbsIndex_r4/Constant  const=2  gui_display_data_type=Fixed-point  arith_type=Unsigned  n_bits=3  bin_pt=0  preci_type=Single  exp_width=8  frac_width=24  explicit_period=on  period=1  equ=P=C  opselect=C  inp2=PCIN>>17  opr=+  inp1=P  carry=CIN  dbl_ovrd=off  block_type=constant
  Constant3 : xbsIndex_r4/Constant  const=3  gui_display_data_type=Fixed-point  arith_type=Unsigned  n_bits=3  bin_pt=0  preci_type=Single  exp_width=8  frac_width=24  explicit_period=on  period=1  equ=P=C  opselect=C  inp2=PCIN>>17  opr=+  inp1=P  carry=CIN  dbl_ovrd=off  block_type=constant
  Constant4 : xbsIndex_r4/Constant  const=4  gui_display_data_type=Fixed-point  arith_type=Unsigned  n_bits=3  bin_pt=0  preci_type=Single  exp_width=8  frac_width=24  explicit_period=on  period=1  equ=P=C  opselect=C  inp2=PCIN>>17  opr=+  inp1=P  carry=CIN  dbl_ovrd=off  block_type=constant
  Constant5 : xbsIndex_r4/Constant  const=5  gui_display_data_type=Fixed-point  arith_type=Unsigned  n_bits=3  bin_pt=0  preci_type=Single  exp_width=8  frac_width=24  explicit_period=on  period=1  equ=P=C  opselect=C  inp2=PCIN>>17  opr=+  inp1=P  carry=CIN  dbl_ovrd=off  block_type=constant
  Constant6 : xbsIndex_r4/Constant  const=6  gui_display_data_type=Fixed-point  arith_type=Unsigned  n_bits=3  bin_pt=0  preci_type=Single  exp_width=8  frac_width=24  explicit_period=on  period=1  equ=P=C  opselect=C  inp2=PCIN>>17  opr=+  inp1=P  carry=CIN  dbl_ovrd=off  block_type=constant
  Constant7 : xbsIndex_r4/Constant  const=7  gui_display_data_type=Fixed-point  arith_type=Unsigned  n_bits=3  bin_pt=0  preci_type=Single  exp_width=8  frac_width=24  explicit_period=on  period=1  equ=P=C  opselect=C  inp2=PCIN>>17  opr=+  inp1=P  carry=CIN  dbl_ovrd=off  block_type=constant
  Logical{1..9} (9 alike) : xbsIndex_r4/Logical  logical_function=AND  inputs=2  en=off  latency=0  precision=Full  arith_type=Unsigned  n_bits=16  bin_pt=0  align_bp=on  dbl_ovrd=off  block_type=logical
  Relational{,1..7} (8 alike) : xbsIndex_r4/Relational  mode=a=b  en=off  latency=0  dbl_ovrd=off  block_type=relational
  Out0 : Outport
  Out1 : Outport  Port=2
  Out2 : Outport  Port=3
  Out3 : Outport  Port=4
  Out4 : Outport  Port=5
  Out5 : Outport  Port=6
  Out6 : Outport  Port=7
  Out7 : Outport  Port=8
  wires:
  Constant4/1 -> Relational4/1
  Constant5/1 -> Relational5/1
  Constant6/1 -> Relational6/1
  Constant1/1 -> Relational1/1
  Relational1/1 -> Logical1/1
  Relational2/1 -> Logical2/1
  Relational/1 -> Logical8/1
  Relational6/1 -> Logical6/1
  Relational3/1 -> Logical3/1
  Relational5/1 -> Logical5/1
  Relational4/1 -> Logical4/1
  Addr/1 -> Relational7/2, Relational6/2, Relational5/2, Relational4/2, Relational3/2, Relational2/2, Relational1/2, Relational/2
  Constant/1 -> Relational/1
  Constant2/1 -> Relational2/1
  Constant3/1 -> Relational3/1
  Constant7/1 -> Relational7/1
  Relational7/1 -> Logical7/1
  Logical9/1 -> Logical8/2, Logical1/2, Logical2/2, Logical3/2, Logical4/2, Logical5/2, Logical7/2, Logical6/2
  Logical8/1 -> Out0/1
  Logical1/1 -> Out1/1
  Logical2/1 -> Out2/1
  Logical3/1 -> Out3/1
  Logical4/1 -> Out4/1
  Logical5/1 -> Out5/1
  Logical6/1 -> Out6/1
  Logical7/1 -> Out7/1
  BitIn/1 -> Logical9/1
  en/1 -> Logical9/2

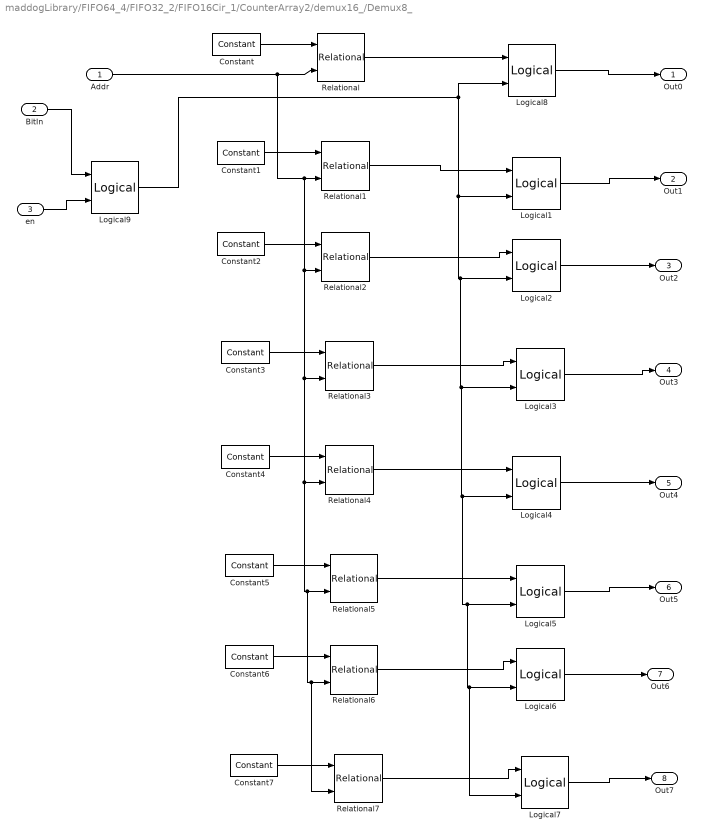
== system maddogLibrary/FIFO64_4/FIFO32_2/FIFO16Cir_1/CounterArray2/demux16_/Demux8_ ==
  Addr : Inport
  BitIn : Inport  Port=2
  en : Inport  Port=3
  Constant : xbsIndex_r4/Constant  const=0  gui_display_data_type=Fixed-point  arith_type=Unsigned  n_bits=3  bin_pt=0  preci_type=Single  exp_width=8  frac_width=24  explicit_period=on  period=1  equ=P=C  opselect=C  inp2=PCIN>>17  opr=+  inp1=P  carry=CIN  dbl_ovrd=off  block_type=constant
  Constant1 : xbsIndex_r4/Constant  const=1  gui_display_data_type=Fixed-point  arith_type=Unsigned  n_bits=3  bin_pt=0  preci_type=Single  exp_width=8  frac_width=24  explicit_period=on  period=1  equ=P=C  opselect=C  inp2=PCIN>>17  opr=+  inp1=P  carry=CIN  dbl_ovrd=off  block_type=constant
  Constant2 : xbsIndex_r4/Constant  const=2  gui_display_data_type=Fixed-point  arith_type=Unsigned  n_bits=3  bin_pt=0  preci_type=Single  exp_width=8  frac_width=24  explicit_period=on  period=1  equ=P=C  opselect=C  inp2=PCIN>>17  opr=+  inp1=P  carry=CIN  dbl_ovrd=off  block_type=constant
  Constant3 : xbsIndex_r4/Constant  const=3  gui_display_data_type=Fixed-point  arith_type=Unsigned  n_bits=3  bin_pt=0  preci_type=Single  exp_width=8  frac_width=24  explicit_period=on  period=1  equ=P=C  opselect=C  inp2=PCIN>>17  opr=+  inp1=P  carry=CIN  dbl_ovrd=off  block_type=constant
  Constant4 : xbsIndex_r4/Constant  const=4  gui_display_data_type=Fixed-point  arith_type=Unsigned  n_bits=3  bin_pt=0  preci_type=Single  exp_width=8  frac_width=24  explicit_period=on  period=1  equ=P=C  opselect=C  inp2=PCIN>>17  opr=+  inp1=P  carry=CIN  dbl_ovrd=off  block_type=constant
  Constant5 : xbsIndex_r4/Constant  const=5  gui_display_data_type=Fixed-point  arith_type=Unsigned  n_bits=3  bin_pt=0  preci_type=Single  exp_width=8  frac_width=24  explicit_period=on  period=1  equ=P=C  opselect=C  inp2=PCIN>>17  opr=+  inp1=P  carry=CIN  dbl_ovrd=off  block_type=constant
  Constant6 : xbsIndex_r4/Constant  const=6  gui_display_data_type=Fixed-point  arith_type=Unsigned  n_bits=3  bin_pt=0  preci_type=Single  exp_width=8  frac_width=24  explicit_period=on  period=1  equ=P=C  opselect=C  inp2=PCIN>>17  opr=+  inp1=P  carry=CIN  dbl_ovrd=off  block_type=constant
  Constant7 : xbsIndex_r4/Constant  const=7  gui_display_data_type=Fixed-point  arith_type=Unsigned  n_bits=3  bin_pt=0  preci_type=Single  exp_width=8  frac_width=24  explicit_period=on  period=1  equ=P=C  opselect=C  inp2=PCIN>>17  opr=+  inp1=P  carry=CIN  dbl_ovrd=off  block_type=constant
  Logical{1..9} (9 alike) : xbsIndex_r4/Logical  logical_function=AND  inputs=2  en=off  latency=0  precision=Full  arith_type=Unsigned  n_bits=16  bin_pt=0  align_bp=on  dbl_ovrd=off  block_type=logical
  Relational{,1..7} (8 alike) : xbsIndex_r4/Relational  mode=a=b  en=off  latency=0  dbl_ovrd=off  block_type=relational
  Out0 : Outport
  Out1 : Outport  Port=2
  Out2 : Outport  Port=3
  Out3 : Outport  Port=4
  Out4 : Outport  Port=5
  Out5 : Outport  Port=6
  Out6 : Outport  Port=7
  Out7 : Outport  Port=8
  wires:
  Constant4/1 -> Relational4/1
  Constant5/1 -> Relational5/1
  Constant6/1 -> Relational6/1
  Constant1/1 -> Relational1/1
  Relational1/1 -> Logical1/1
  Relational2/1 -> Logical2/1
  Relational/1 -> Logical8/1
  Relational6/1 -> Logical6/1
  Relational3/1 -> Logical3/1
  Relational5/1 -> Logical5/1
  Relational4/1 -> Logical4/1
  Addr/1 -> Relational7/2, Relational6/2, Relational5/2, Relational4/2, Relational3/2, Relational2/2, Relational1/2, Relational/2
  Constant/1 -> Relational/1
  Constant2/1 -> Relational2/1
  Constant3/1 -> Relational3/1
  Constant7/1 -> Relational7/1
  Relational7/1 -> Logical7/1
  Logical9/1 -> Logical8/2, Logical7/2, Logical6/2, Logical5/2, Logical4/2, Logical3/2, Logical2/2, Logical1/2
  Logical8/1 -> Out0/1
  Logical1/1 -> Out1/1
  Logical2/1 -> Out2/1
  Logical3/1 -> Out3/1
  Logical4/1 -> Out4/1
  Logical5/1 -> Out5/1
  Logical6/1 -> Out6/1
  Logical7/1 -> Out7/1
  BitIn/1 -> Logical9/1
  en/1 -> Logical9/2

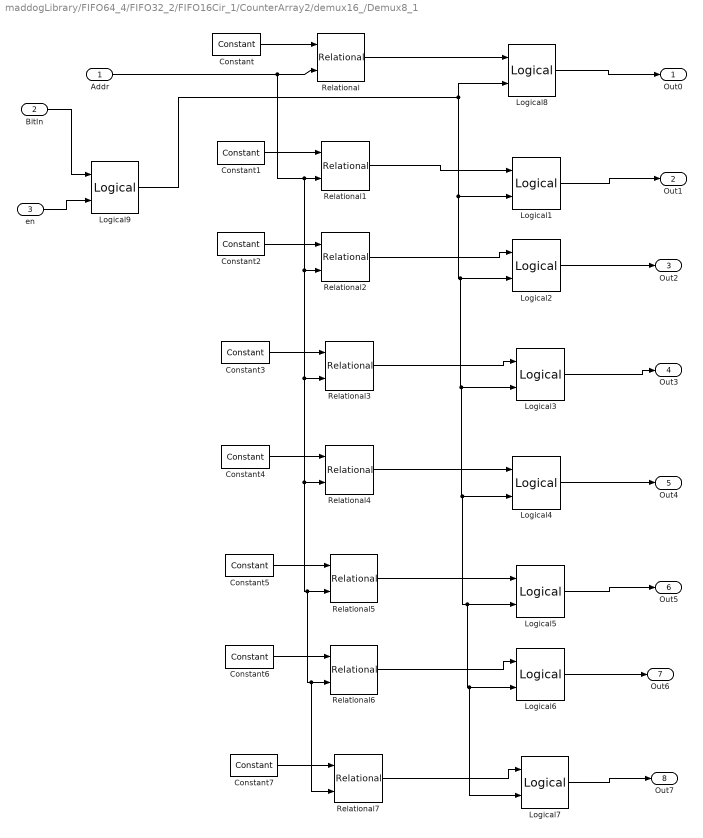
== system maddogLibrary/FIFO64_4/FIFO32_2/FIFO16Cir_1/CounterArray2/demux16_/Demux8_1 ==
  Addr : Inport
  BitIn : Inport  Port=2
  en : Inport  Port=3
  Constant : xbsIndex_r4/Constant  const=0  gui_display_data_type=Fixed-point  arith_type=Unsigned  n_bits=3  bin_pt=0  preci_type=Single  exp_width=8  frac_width=24  explicit_period=on  period=1  equ=P=C  opselect=C  inp2=PCIN>>17  opr=+  inp1=P  carry=CIN  dbl_ovrd=off  block_type=constant
  Constant1 : xbsIndex_r4/Constant  const=1  gui_display_data_type=Fixed-point  arith_type=Unsigned  n_bits=3  bin_pt=0  preci_type=Single  exp_width=8  frac_width=24  explicit_period=on  period=1  equ=P=C  opselect=C  inp2=PCIN>>17  opr=+  inp1=P  carry=CIN  dbl_ovrd=off  block_type=constant
  Constant2 : xbsIndex_r4/Constant  const=2  gui_display_data_type=Fixed-point  arith_type=Unsigned  n_bits=3  bin_pt=0  preci_type=Single  exp_width=8  frac_width=24  explicit_period=on  period=1  equ=P=C  opselect=C  inp2=PCIN>>17  opr=+  inp1=P  carry=CIN  dbl_ovrd=off  block_type=constant
  Constant3 : xbsIndex_r4/Constant  const=3  gui_display_data_type=Fixed-point  arith_type=Unsigned  n_bits=3  bin_pt=0  preci_type=Single  exp_width=8  frac_width=24  explicit_period=on  period=1  equ=P=C  opselect=C  inp2=PCIN>>17  opr=+  inp1=P  carry=CIN  dbl_ovrd=off  block_type=constant
  Constant4 : xbsIndex_r4/Constant  const=4  gui_display_data_type=Fixed-point  arith_type=Unsigned  n_bits=3  bin_pt=0  preci_type=Single  exp_width=8  frac_width=24  explicit_period=on  period=1  equ=P=C  opselect=C  inp2=PCIN>>17  opr=+  inp1=P  carry=CIN  dbl_ovrd=off  block_type=constant
  Constant5 : xbsIndex_r4/Constant  const=5  gui_display_data_type=Fixed-point  arith_type=Unsigned  n_bits=3  bin_pt=0  preci_type=Single  exp_width=8  frac_width=24  explicit_period=on  period=1  equ=P=C  opselect=C  inp2=PCIN>>17  opr=+  inp1=P  carry=CIN  dbl_ovrd=off  block_type=constant
  Constant6 : xbsIndex_r4/Constant  const=6  gui_display_data_type=Fixed-point  arith_type=Unsigned  n_bits=3  bin_pt=0  preci_type=Single  exp_width=8  frac_width=24  explicit_period=on  period=1  equ=P=C  opselect=C  inp2=PCIN>>17  opr=+  inp1=P  carry=CIN  dbl_ovrd=off  block_type=constant
  Constant7 : xbsIndex_r4/Constant  const=7  gui_display_data_type=Fixed-point  arith_type=Unsigned  n_bits=3  bin_pt=0  preci_type=Single  exp_width=8  frac_width=24  explicit_period=on  period=1  equ=P=C  opselect=C  inp2=PCIN>>17  opr=+  inp1=P  carry=CIN  dbl_ovrd=off  block_type=constant
  Logical{1..9} (9 alike) : xbsIndex_r4/Logical  logical_function=AND  inputs=2  en=off  latency=0  precision=Full  arith_type=Unsigned  n_bits=16  bin_pt=0  align_bp=on  dbl_ovrd=off  block_type=logical
  Relational{,1..7} (8 alike) : xbsIndex_r4/Relational  mode=a=b  en=off  latency=0  dbl_ovrd=off  block_type=relational
  Out0 : Outport
  Out1 : Outport  Port=2
  Out2 : Outport  Port=3
  Out3 : Outport  Port=4
  Out4 : Outport  Port=5
  Out5 : Outport  Port=6
  Out6 : Outport  Port=7
  Out7 : Outport  Port=8
  wires:
  Constant4/1 -> Relational4/1
  Constant5/1 -> Relational5/1
  Constant6/1 -> Relational6/1
  Constant1/1 -> Relational1/1
  Relational1/1 -> Logical1/1
  Relational2/1 -> Logical2/1
  Relational/1 -> Logical8/1
  Relational6/1 -> Logical6/1
  Relational3/1 -> Logical3/1
  Relational5/1 -> Logical5/1
  Relational4/1 -> Logical4/1
  Addr/1 -> Relational7/2, Relational6/2, Relational5/2, Relational4/2, Relational3/2, Relational2/2, Relational1/2, Relational/2
  Constant/1 -> Relational/1
  Constant2/1 -> Relational2/1
  Constant3/1 -> Relational3/1
  Constant7/1 -> Relational7/1
  Relational7/1 -> Logical7/1
  Logical9/1 -> Logical8/2, Logical7/2, Logical6/2, Logical5/2, Logical4/2, Logical3/2, Logical2/2, Logical1/2
  Logical8/1 -> Out0/1
  Logical1/1 -> Out1/1
  Logical2/1 -> Out2/1
  Logical3/1 -> Out3/1
  Logical4/1 -> Out4/1
  Logical5/1 -> Out5/1
  Logical6/1 -> Out6/1
  Logical7/1 -> Out7/1
  BitIn/1 -> Logical9/1
  en/1 -> Logical9/2
